simulink model "ControlSystemExercise1"  (R2019b)
settings: Solver=VariableStepAuto  StartTime=0.0  StopTime=15  RelTol=1e-8  AbsTol=1e-9
libraries: simulink x2
settings Model: Creator=19398  LastModifiedBy=19398

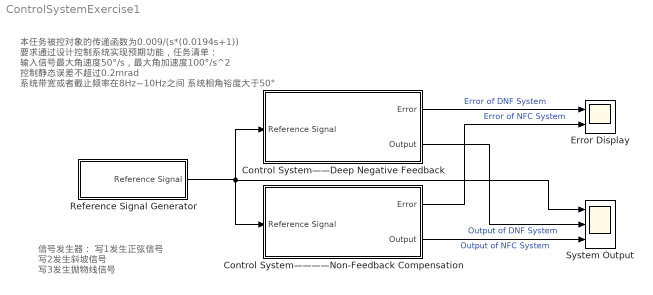
== system ControlSystemExercise1 ==
  note: 信号发生器：
      | 写1发生正弦信号
      | 写2发生斜坡信号
      | 写3发生抛物线信号
  note: 本任务被控对象的传递函数为0.009/(s*(0.0194s+1))
      | 要求通过设计控制系统实现预期功能，任务清单：
      | 输入信号最大角速度50°/s，最大角加速度100°/s^2
      | 控制静态误差不超过0.2mrad
      | 系统带宽或者截止频率在8Hz~10Hz之间
      | 系统相角裕度大于50°
  Control System——Deep Negative Feedback : Subsystem
  Control System————Non-Feedback Compensation : Subsystem
  Error Display : Scope  NumInputPorts=2
  Reference Signal Generator : Subsystem  mask{SignalIndex=1}
      mask prompts: SignalIndex "Select typical type of Reference signal"
  System Output : Scope  NumInputPorts=3
  wires:
  Control System——Deep Negative Feedback/1(Error) -> Error Display/1  "Error of DNF System"
  Control System————Non-Feedback Compensation/1(Error) -> Error Display/2  "Error of NFC System"
  Control System——Deep Negative Feedback/2(Output) -> System Output/2  "Output of DNF System"
  Control System————Non-Feedback Compensation/2(Output) -> System Output/3  "Output of NFC System"
  Reference Signal Generator/1(Reference Signal) -> Control System————Non-Feedback Compensation/1(Reference Signal), System Output/1, Control System——Deep Negative Feedback/1(Reference Signal)

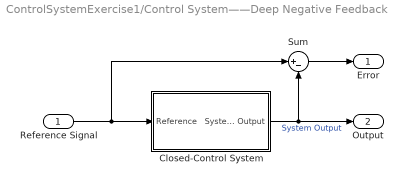
== system ControlSystemExercise1/Control System——Deep Negative Feedback ==
  Reference Signal : Inport
  Closed-Control System : Subsystem
  Sum : Sum  Inputs=|+-
  Error : Outport
  Output : Outport  Port=2
  wires:
  Sum/1 -> Error/1
  Reference Signal/1 -> Sum/1, Closed-Control System/1(Reference)
  Closed-Control System/1(System Output) -> Output/1, Sum/2  "System Output"

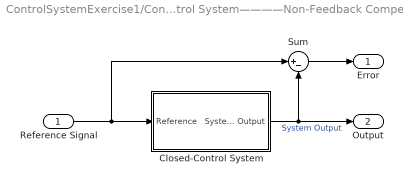
== system ControlSystemExercise1/Control System————Non-Feedback Compensation ==
  Reference Signal : Inport
  Closed-Control System : Subsystem
  Sum : Sum  Inputs=|+-
  Error : Outport
  Output : Outport  Port=2
  wires:
  Sum/1 -> Error/1
  Reference Signal/1 -> Sum/1, Closed-Control System/1(Reference)
  Closed-Control System/1(System Output) -> Output/1, Sum/2  "System Output"

== system ControlSystemExercise1/Reference Signal Generator ==
  Reference Signal Generator : Subsystem
  Signal Select : Constant  Value=SignalIndex
  Reference Signal : Outport
  wires:
  Signal Select/1 -> Reference Signal Generator/1(Select Port)
  Reference Signal Generator/1(Reference) -> Reference Signal/1  "Reference"

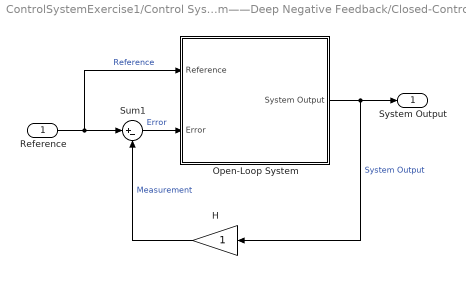
== system ControlSystemExercise1/Control System——Deep Negative Feedback/Closed-Control System ==
  Reference : Inport
  H : Gain
  Open-Loop System : Subsystem
  Sum1 : Sum  Inputs=|+-
  System Output : Outport
  wires:
  Reference/1 -> Open-Loop System/1(Reference), Sum1/1  "Reference"
  H/1 -> Sum1/2  "Measurement"
  Open-Loop System/1(System Output) -> System Output/1, H/1  "System Output"
  Sum1/1 -> Open-Loop System/2(Error)  "Error"

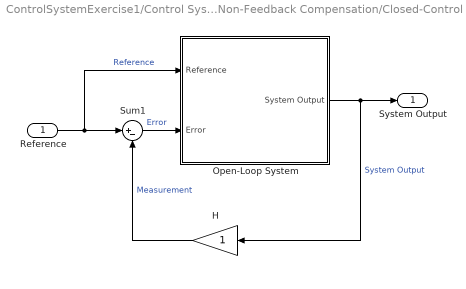
== system ControlSystemExercise1/Control System————Non-Feedback Compensation/Closed-Control System ==
  Reference : Inport
  H : Gain
  Open-Loop System : Subsystem
  Sum1 : Sum  Inputs=|+-
  System Output : Outport
  wires:
  Reference/1 -> Open-Loop System/1(Reference), Sum1/1  "Reference"
  H/1 -> Sum1/2  "Measurement"
  Open-Loop System/1(System Output) -> System Output/1, H/1  "System Output"
  Sum1/1 -> Open-Loop System/2(Error)  "Error"

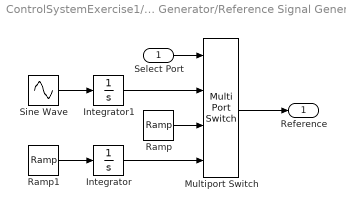
== system ControlSystemExercise1/Reference Signal Generator/Reference Signal Generator ==
  Select Port : Inport
  Integrator : Integrator
  Integrator1 : Integrator
  Multiport Switch : MultiPortSwitch
  Ramp : simulink/Sources/Ramp  slope=50  start=0  InitialOutput=0
  Ramp1 : simulink/Sources/Ramp  slope=100  start=0  InitialOutput=0
  Sine Wave : Sin  Amplitude=50  Frequency=2  SampleTime=0
  Reference : Outport
  wires:
  Select Port/1 -> Multiport Switch/1
  Multiport Switch/1 -> Reference/1
  Sine Wave/1 -> Integrator1/1
  Ramp/1 -> Multiport Switch/3
  Ramp1/1 -> Integrator/1
  Integrator/1 -> Multiport Switch/4
  Integrator1/1 -> Multiport Switch/2

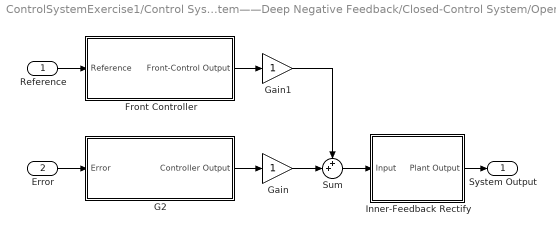
== system ControlSystemExercise1/Control System——Deep Negative Feedback/Closed-Control System/Open-Loop System ==
  Reference : Inport
  Error : Inport  Port=2
  Front Controller : Subsystem
  G2 : Subsystem
  Gain : Gain
  Gain1 : Gain
  Inner-Feedback Rectify : Subsystem
  Sum : Sum  Inputs=++|
  System Output : Outport
  wires:
  Sum/1 -> Inner-Feedback Rectify/1(Input)
  Gain/1 -> Sum/2
  Reference/1 -> Front Controller/1(Reference)
  Inner-Feedback Rectify/1(Plant Output) -> System Output/1
  Error/1 -> G2/1(Error)
  G2/1(Controller Output) -> Gain/1
  Gain1/1 -> Sum/1
  Front Controller/1(Front-Control Output) -> Gain1/1

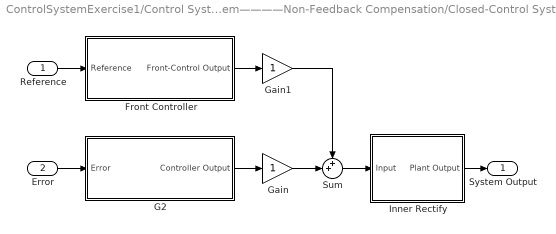
== system ControlSystemExercise1/Control System————Non-Feedback Compensation/Closed-Control System/Open-Loop System ==
  Reference : Inport
  Error : Inport  Port=2
  Front Controller : Subsystem
  G2 : Subsystem
  Gain : Gain
  Gain1 : Gain
  Inner Rectify : Subsystem
  Sum : Sum  Inputs=++|
  System Output : Outport
  wires:
  Sum/1 -> Inner Rectify/1(Input)
  Gain/1 -> Sum/2
  Reference/1 -> Front Controller/1(Reference)
  Inner Rectify/1(Plant Output) -> System Output/1
  Error/1 -> G2/1(Error)
  G2/1(Controller Output) -> Gain/1
  Gain1/1 -> Sum/1
  Front Controller/1(Front-Control Output) -> Gain1/1

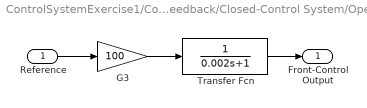
== system ControlSystemExercise1/Control System——Deep Negative Feedback/Closed-Control System/Open-Loop System/Front Controller ==
  Reference : Inport
  G3 : Gain  Gain=100
  Transfer Fcn : TransferFcn  Denominator=[0.002 1]
  Front-Control Output : Outport
  wires:
  Reference/1 -> G3/1
  G3/1 -> Transfer Fcn/1
  Transfer Fcn/1 -> Front-Control Output/1

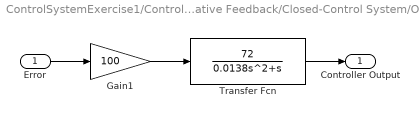
== system ControlSystemExercise1/Control System——Deep Negative Feedback/Closed-Control System/Open-Loop System/G2 ==
  Error : Inport
  Gain1 : Gain  Gain=100
  Transfer Fcn : TransferFcn  Numerator=[72]  Denominator=[0.0138 1 0]
  Controller Output : Outport
  wires:
  Error/1 -> Gain1/1
  Gain1/1 -> Transfer Fcn/1
  Transfer Fcn/1 -> Controller Output/1

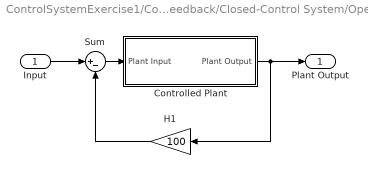
== system ControlSystemExercise1/Control System——Deep Negative Feedback/Closed-Control System/Open-Loop System/Inner-Feedback Rectify ==
  Input : Inport
  Controlled Plant : Subsystem
  H1 : Gain  Gain=100
  Sum : Sum  Inputs=|+-
  Plant Output : Outport
  wires:
  Controlled Plant/1(Plant Output) -> H1/1, Plant Output/1
  H1/1 -> Sum/2
  Sum/1 -> Controlled Plant/1(Plant Input)
  Input/1 -> Sum/1

== system ControlSystemExercise1/Control System————Non-Feedback Compensation/Closed-Control System/Open-Loop System/Front Controller ==
  Reference : Inport
  Transfer Fcn1 : TransferFcn  Numerator=[0.0194 1 0]  Denominator=conv([0.001 1],[0.001 1])
  Front-Control Output : Outport
  wires:
  Transfer Fcn1/1 -> Front-Control Output/1
  Reference/1 -> Transfer Fcn1/1

== system ControlSystemExercise1/Control System————Non-Feedback Compensation/Closed-Control System/Open-Loop System/G2 ==
  Error : Inport
  Gain1 : Gain  Gain=72
  Transfer Fcn : TransferFcn  Numerator=[0.0194 1]  Denominator=[0.0138 1]
  Controller Output : Outport
  wires:
  Error/1 -> Gain1/1
  Gain1/1 -> Transfer Fcn/1
  Transfer Fcn/1 -> Controller Output/1

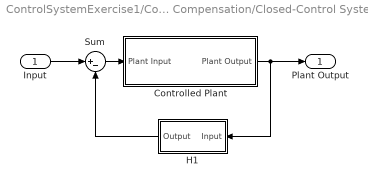
== system ControlSystemExercise1/Control System————Non-Feedback Compensation/Closed-Control System/Open-Loop System/Inner Rectify ==
  Input : Inport
  Controlled Plant : Subsystem
  H1 : Subsystem
  Sum : Sum  Inputs=|+-
  Plant Output : Outport
  wires:
  Controlled Plant/1(Plant Output) -> H1/1(Input), Plant Output/1
  Sum/1 -> Controlled Plant/1(Plant Input)
  Input/1 -> Sum/1
  H1/1(Output) -> Sum/2

== system ControlSystemExercise1/Control System——Deep Negative Feedback/Closed-Control System/Open-Loop System/Inner-Feedback Rectify/Controlled Plant ==
  Plant Input : Inport
  G2 : Subsystem
  Plant : Subsystem
  Plant Output : Outport
  wires:
  Plant/1(System Output) -> Plant Output/1
  Plant Input/1 -> G2/1(Input)
  G2/1(Output) -> Plant/1(Controlled Variable)

== system ControlSystemExercise1/Control System————Non-Feedback Compensation/Closed-Control System/Open-Loop System/Inner Rectify/Controlled Plant ==
  Plant Input : Inport
  G1 : Gain  Gain=112
  Plant : Subsystem
  Plant Output : Outport
  wires:
  Plant/1(System Output) -> Plant Output/1
  Plant Input/1 -> G1/1
  G1/1 -> Plant/1(Controlled Variable)

== system ControlSystemExercise1/Control System————Non-Feedback Compensation/Closed-Control System/Open-Loop System/Inner Rectify/H1 ==
  Input : Inport
  Gain : Gain  Gain=0
  Output : Outport
  wires:
  Gain/1 -> Output/1
  Input/1 -> Gain/1

== system ControlSystemExercise1/Control System——Deep Negative Feedback/Closed-Control System/Open-Loop System/Inner-Feedback Rectify/Controlled Plant/G2 ==
  Input : Inport
  Transfer Fcn : TransferFcn  Numerator=[0.02 1]  Denominator=[0.002 1]
  gain : Gain  Gain=1800
  Output : Outport
  wires:
  gain/1 -> Transfer Fcn/1
  Input/1 -> gain/1
  Transfer Fcn/1 -> Output/1

== system ControlSystemExercise1/Control System——Deep Negative Feedback/Closed-Control System/Open-Loop System/Inner-Feedback Rectify/Controlled Plant/Plant ==
  Controlled Variable : Inport
  Gain : Gain  Gain=0.5
  Object : TransferFcn  Numerator=[0.018]  Denominator=[0.0194 1 0]
  System Output : Outport
  wires:
  Object/1 -> Gain/1
  Controlled Variable/1 -> Object/1
  Gain/1 -> System Output/1

== system ControlSystemExercise1/Control System————Non-Feedback Compensation/Closed-Control System/Open-Loop System/Inner Rectify/Controlled Plant/Plant ==
  Controlled Variable : Inport
  Gain : Gain  Gain=0.5
  Object : TransferFcn  Numerator=[0.018]  Denominator=[0.0194 1 0]
  System Output : Outport
  wires:
  Object/1 -> Gain/1
  Controlled Variable/1 -> Object/1
  Gain/1 -> System Output/1
